simulink model "do_feedforward_cascade"  (R2024b)
settings: Solver=ode45  StartTime=0.0  StopTime=2400  RelTol=1e-3
libraries: slpidlib x2
settings Model: Creator=Administrator  LastModifiedBy=Administrator

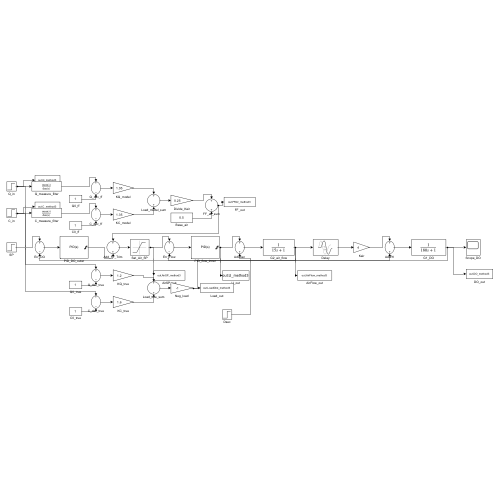
[thumbnail: Simulink's stored preview of the top-level diagram]
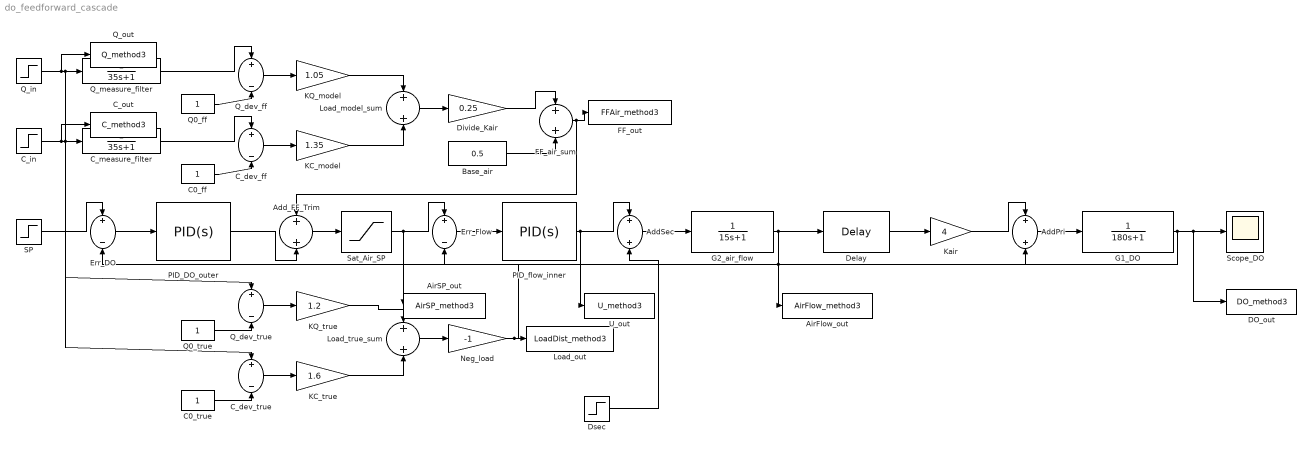
== system do_feedforward_cascade ==
  AddPri : Sum
  AddSec : Sum
  Add_FF_Trim : Sum
  AirFlow_out : ToWorkspace  VariableName=AirFlow_method3  SaveFormat=Structure With Time  SampleTime=-1
  AirSP_out : ToWorkspace  VariableName=AirSP_method3  SaveFormat=Structure With Time  SampleTime=-1
  Base_air : Constant  Value=0.5
  C0_ff : Constant
  C0_true : Constant
  C_dev_ff : Sum  Inputs=+-
  C_dev_true : Sum  Inputs=+-
  C_in : Step  Time=1200  Before=1  After=1.4  SampleTime=0
  C_measure_filter : TransferFcn  Denominator=[35 1]
  C_out : ToWorkspace  VariableName=C_method3  SaveFormat=Structure With Time  SampleTime=-1
  DO_out : ToWorkspace  VariableName=DO_method3  SaveFormat=Structure With Time  SampleTime=-1
  Delay : TransportDelay  DelayTime=30  BufferSize=8192
  Divide_Kair : Gain  Gain=0.25
  Dsec : Step  Time=1200  After=0  SampleTime=0
  Err_DO : Sum  Inputs=+-
  Err_Flow : Sum  Inputs=+-
  FF_air_sum : Sum
  FF_out : ToWorkspace  VariableName=FFAir_method3  SaveFormat=Structure With Time  SampleTime=-1
  G1_DO : TransferFcn  Denominator=[180 1]
  G2_air_flow : TransferFcn  Denominator=[15 1]
  KC_model : Gain  Gain=1.35
  KC_true : Gain  Gain=1.6
  KQ_model : Gain  Gain=1.05
  KQ_true : Gain  Gain=1.2
  Kair : Gain  Gain=4
  Load_model_sum : Sum
  Load_out : ToWorkspace  VariableName=LoadDist_method3  SaveFormat=Structure With Time  SampleTime=-1
  Load_true_sum : Sum
  Neg_load : Gain  Gain=-1
  PID_DO_outer : slpidlib/PID Controller  Controller=PID  Form=Parallel  TimeDomain=Continuous-time  UseExternalTs=off  SampleTime=-1  IntegratorMethod=Forward Euler  FilterMethod=Forward Euler  ControllerParametersSource=internal  P=0.26  I=0.0015  UseKiTs=off  D=8  UseExternalDerivativeSource=off  N=2  UseFilter=on  TunerSelectOption=Transfer Function Based (PID Tuner App)  InitialConditionSource=internal  InitialConditionForIntegrator=0  InitialConditionForFilter=0  DifferentiatorICPrevScaledInput=0  ExternalReset=none  TrackingMode=off  Kt=1  LimitOutput=on  SatLimitsSource=internal  UpperSaturationLimit=0.25  LowerSaturationLimit=-0.25  LinearizeAsGain=on  AntiWindupMode=clamping  Kb=1  LimitIntegrator=off  UpperIntegratorSaturationLimit=inf  LowerIntegratorSaturationLimit=-inf  POutMin=[]  POutMax=[]  IOutMin=[]  IOutMax=[]  DOutMin=[]  DOutMax=[]  NOutMin=[]  NOutMax=[]  SumOutMin=[]  SumOutMax=[]  SaturationOutMin=[]  SaturationOutMax=[]  PParamMin=[]  PParamMax=[]  IParamMin=[]  IParamMax=[]  DParamMin=[]  DParamMax=[]  NParamMin=[]  NParamMax=[]  KbParamMin=[]  KbParamMax=[]  KtParamMin=[]  KtParamMax=[]  KbOutMin=[]  KbOutMax=[]  KtOutMin=[]  KtOutMax=[]  IntegratorOutMin=[]  IntegratorOutMax=[]  FilterOutMin=[]  FilterOutMax=[]  SumI1OutMin=[]  SumI1OutMax=[]  SumI2OutMin=[]  SumI2OutMax=[]  SumI3OutMin=[]  SumI3OutMax=[]  SumI4OutMin=[]  SumI4OutMax=[]  SumDOutMin=[]  SumDOutMax=[]  DifferentiatorOutMin=[]  DifferentiatorOutMax=[]  FilterDiffOutCoefMin=[]  FilterDiffOutCoefMax=[]  ReciprocalOutMin=[]  ReciprocalOutMax=[]  SumDenOutMin=[]  SumDenOutMax=[]  SumNumOutMin=[]  SumNumOutMax=[]  DivideOutMin=[]  DivideOutMax=[]  UdiffTsProdOutMin=[]  UdiffTsProdOutMax=[]  NTsProdOutMin=[]  NTsProdOutMax=[]  UintegralTsProdOutMin=[]  UintegralTsProdOutMax=[]  UngainTsProdOutMin=[]  UngainTsProdOutMax=[]  ClampingZeroOutDataTypeStr=Inherit: Inherit via back propagation  ClampingZeroOutMin=[]  ClampingZeroOutMax=[]  FilterDenConstantOutDataTypeStr=Inherit: Inherit via back propagation  FilterDenConstantOutMin=[]  FilterDenConstantOutMax=[]  PCopyOutDataTypeStr=Inherit: Inherit via back propagation  PCopyOutMin=[]  PCopyOutMax=[]  NCopyOutDataTypeStr=Inherit: Inherit via back propagation  NCopyOutMin=[]  NCopyOutMax=[]  IntegratorContinuousStateAttributes=''  IntegratorStateMustResolveToSignalObject=off  IntegratorRTWStateStorageClass=Auto  FilterContinuousStateAttributes=''  FilterStateMustResolveToSignalObject=off  FilterRTWStateStorageClass=Auto  ParallelPVariant=InternalParameters  IdealPVariant=Disabled  IVariant=InternalParameters  DVariant=InternalParameters  IntegratorVariant=Continuous  SatVariant=Enabled  AWVariant=ContClampingParallel  PCopyVariant=Disabled  TRVariant=Disabled  FdbkBlocksVariant=Forward  IdealPFdbkVariant=Disabled  SatFdbkVariant=Disabled  DerivativeFilterVariant=ContFilter  NVariant=InternalParameters  NCopyVariant=Disabled  FilterICVariant=InternalICsFilter  IntegratorICVariant=InternalICs  ExternalResetVariant=Disabled  TRSumVariant=Passthrough  SumFdbkVariant=Disabled  SumVariant=Sum_PID  TsampFilterVariant=InternalTs  TsampNgainVariant=Passthrough  TsampIntegralVariant=Disabled_SignalSpec  ExternalSaturationOutDataTypeStr=Inherit: Same as second input  DerivativeSourceVariant=ErrorSignal  PreIntVariant=InternalPreInt
  PID_flow_inner : slpidlib/PID Controller  Controller=PID  Form=Parallel  TimeDomain=Continuous-time  UseExternalTs=off  SampleTime=-1  IntegratorMethod=Forward Euler  FilterMethod=Forward Euler  ControllerParametersSource=internal  P=4  I=0.6  UseKiTs=off  D=0  UseExternalDerivativeSource=off  N=2  UseFilter=on  TunerSelectOption=Transfer Function Based (PID Tuner App)  InitialConditionSource=internal  InitialConditionForIntegrator=0  InitialConditionForFilter=0  DifferentiatorICPrevScaledInput=0  ExternalReset=none  TrackingMode=off  Kt=1  LimitOutput=on  SatLimitsSource=internal  UpperSaturationLimit=1  LowerSaturationLimit=0  LinearizeAsGain=on  AntiWindupMode=clamping  Kb=1  LimitIntegrator=off  UpperIntegratorSaturationLimit=inf  LowerIntegratorSaturationLimit=-inf  POutMin=[]  POutMax=[]  IOutMin=[]  IOutMax=[]  DOutMin=[]  DOutMax=[]  NOutMin=[]  NOutMax=[]  SumOutMin=[]  SumOutMax=[]  SaturationOutMin=[]  SaturationOutMax=[]  PParamMin=[]  PParamMax=[]  IParamMin=[]  IParamMax=[]  DParamMin=[]  DParamMax=[]  NParamMin=[]  NParamMax=[]  KbParamMin=[]  KbParamMax=[]  KtParamMin=[]  KtParamMax=[]  KbOutMin=[]  KbOutMax=[]  KtOutMin=[]  KtOutMax=[]  IntegratorOutMin=[]  IntegratorOutMax=[]  FilterOutMin=[]  FilterOutMax=[]  SumI1OutMin=[]  SumI1OutMax=[]  SumI2OutMin=[]  SumI2OutMax=[]  SumI3OutMin=[]  SumI3OutMax=[]  SumI4OutMin=[]  SumI4OutMax=[]  SumDOutMin=[]  SumDOutMax=[]  DifferentiatorOutMin=[]  DifferentiatorOutMax=[]  FilterDiffOutCoefMin=[]  FilterDiffOutCoefMax=[]  ReciprocalOutMin=[]  ReciprocalOutMax=[]  SumDenOutMin=[]  SumDenOutMax=[]  SumNumOutMin=[]  SumNumOutMax=[]  DivideOutMin=[]  DivideOutMax=[]  UdiffTsProdOutMin=[]  UdiffTsProdOutMax=[]  NTsProdOutMin=[]  NTsProdOutMax=[]  UintegralTsProdOutMin=[]  UintegralTsProdOutMax=[]  UngainTsProdOutMin=[]  UngainTsProdOutMax=[]  ClampingZeroOutDataTypeStr=Inherit: Inherit via back propagation  ClampingZeroOutMin=[]  ClampingZeroOutMax=[]  FilterDenConstantOutDataTypeStr=Inherit: Inherit via back propagation  FilterDenConstantOutMin=[]  FilterDenConstantOutMax=[]  PCopyOutDataTypeStr=Inherit: Inherit via back propagation  PCopyOutMin=[]  PCopyOutMax=[]  NCopyOutDataTypeStr=Inherit: Inherit via back propagation  NCopyOutMin=[]  NCopyOutMax=[]  IntegratorContinuousStateAttributes=''  IntegratorStateMustResolveToSignalObject=off  IntegratorRTWStateStorageClass=Auto  FilterContinuousStateAttributes=''  FilterStateMustResolveToSignalObject=off  FilterRTWStateStorageClass=Auto  ParallelPVariant=InternalParameters  IdealPVariant=Disabled  IVariant=InternalParameters  DVariant=InternalParameters  IntegratorVariant=Continuous  SatVariant=Enabled  AWVariant=ContClampingParallel  PCopyVariant=Disabled  TRVariant=Disabled  FdbkBlocksVariant=Forward  IdealPFdbkVariant=Disabled  SatFdbkVariant=Disabled  DerivativeFilterVariant=ContFilter  NVariant=InternalParameters  NCopyVariant=Disabled  FilterICVariant=InternalICsFilter  IntegratorICVariant=InternalICs  ExternalResetVariant=Disabled  TRSumVariant=Passthrough  SumFdbkVariant=Disabled  SumVariant=Sum_PID  TsampFilterVariant=InternalTs  TsampNgainVariant=Passthrough  TsampIntegralVariant=Disabled_SignalSpec  ExternalSaturationOutDataTypeStr=Inherit: Same as second input  DerivativeSourceVariant=ErrorSignal  PreIntVariant=InternalPreInt
  Q0_ff : Constant
  Q0_true : Constant
  Q_dev_ff : Sum  Inputs=+-
  Q_dev_true : Sum  Inputs=+-
  Q_in : Step  Time=1200  Before=1  After=1.2  SampleTime=0
  Q_measure_filter : TransferFcn  Denominator=[35 1]
  Q_out : ToWorkspace  VariableName=Q_method3  SaveFormat=Structure With Time  SampleTime=-1
  SP : Step  Time=0  After=2  SampleTime=0
  Sat_Air_SP : Saturate  UpperLimit=1  LowerLimit=0
  Scope_DO : Scope
  U_out : ToWorkspace  VariableName=U_method3  SaveFormat=Structure With Time  SampleTime=-1
  wires:
  SP/1 -> Err_DO/1
  Err_DO/1 -> PID_DO_outer/1
  PID_DO_outer/1 -> Add_FF_Trim/2
  Add_FF_Trim/1 -> Sat_Air_SP/1
  Sat_Air_SP/1 -> Err_Flow/1, AirSP_out/1
  Err_Flow/1 -> PID_flow_inner/1
  PID_flow_inner/1 -> AddSec/1, U_out/1
  Dsec/1 -> AddSec/2
  AddSec/1 -> G2_air_flow/1
  G2_air_flow/1 -> AirFlow_out/1, Err_Flow/2, Delay/1
  Delay/1 -> Kair/1
  Kair/1 -> AddPri/1
  AddPri/1 -> G1_DO/1
  G1_DO/1 -> Scope_DO/1, DO_out/1, Err_DO/2
  Q_in/1 -> Q_measure_filter/1, Q_dev_true/1, Q_out/1
  C_in/1 -> C_measure_filter/1, C_dev_true/1, C_out/1
  Q_measure_filter/1 -> Q_dev_ff/1
  Q0_ff/1 -> Q_dev_ff/2
  C_measure_filter/1 -> C_dev_ff/1
  C0_ff/1 -> C_dev_ff/2
  Q_dev_ff/1 -> KQ_model/1
  C_dev_ff/1 -> KC_model/1
  KQ_model/1 -> Load_model_sum/1
  KC_model/1 -> Load_model_sum/2
  Load_model_sum/1 -> Divide_Kair/1
  Divide_Kair/1 -> FF_air_sum/1
  Base_air/1 -> FF_air_sum/2
  FF_air_sum/1 -> Add_FF_Trim/1, FF_out/1
  Q0_true/1 -> Q_dev_true/2
  C0_true/1 -> C_dev_true/2
  Q_dev_true/1 -> KQ_true/1
  C_dev_true/1 -> KC_true/1
  KQ_true/1 -> Load_true_sum/1
  KC_true/1 -> Load_true_sum/2
  Load_true_sum/1 -> Neg_load/1
  Neg_load/1 -> AddPri/2, Load_out/1
